simulink model "DC"  (R2016b)
settings: Solver=ode4  StartTime=0.0  StopTime=Inf  FixedStep=0.005  RelTol=1e-3
settings Model: Creator=ANTO_  LastModifiedBy=ANTO_
settings DebuggingCC: RootOutportRequireBusObject=error  StrictBusMsg=ErrorOnBusTreatedAsVector
settings HardwareCC: ProdBitPerPointer=32  ProdBitPerSizeT=32  ProdBitPerPtrDiffT=32  ProdLargestAtomicInteger=Long  ProdWordSize=32  ProdHWDeviceType=ARM Compatible->ARM 7
settings RTWCC: SystemTargetFile=NIVeriStand_Linux_ARM_32.tlc  TemplateMakefile=NIVeriStand_Linux_ARM_32.tmf  Description=NI Linux Real-Time ARM (32-bit) Target
settings STFCustomTargetCC: TargetLangStandard=C99 (ISO)  MatFileLogging=on  MATLABClassNameForMDSCustomization=Simulink.SoftwareTarget.TargetSpecificTriggerConfigurationBase  SystemTargetFile=NIVeriStand_Linux_ARM_32.tlc

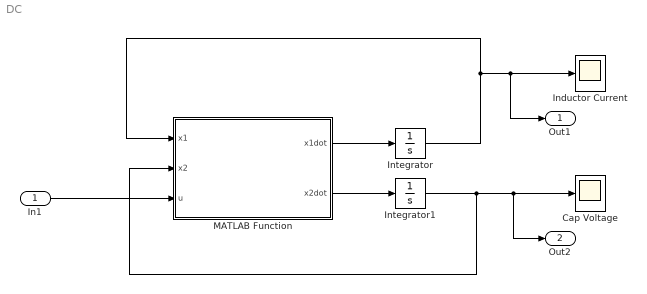
== system DC ==
  In1 : Inport
  Cap Voltage : Scope
  Inductor Current : Scope
  Integrator : Integrator  InitialCondition=0.7
  Integrator1 : Integrator  InitialCondition=5.4
  MATLAB Function : MATLAB Function  TreatAsAtomicUnit=on
  Out1 : Outport
  Out2 : Outport  Port=2
  wires:
  MATLAB Function/1(x1dot) -> Integrator/1
  MATLAB Function/2(x2dot) -> Integrator1/1
  Integrator/1 -> MATLAB Function/1(x1), Out1/1, Inductor Current/1
  Integrator1/1 -> MATLAB Function/2(x2), Out2/1, Cap Voltage/1
  In1/1 -> MATLAB Function/3(u)

== matlab function DC/MATLAB Function ==
  data: x1 input; x2 input; u input; x1dot output; x2dot output
function [x1dot,x2dot] = Boost_DC_converter(x1,x2,u)

  x = [x1;x2];
  r0=1.0;
  vs = 1.0 ;
  rl = 0.05 ;
  rc = rl / 10 ;
  xl = 3.0 ;
  xc = 70.0 ;

  if(u==1)
    A = [ -rl / xl  0 ;  0  (-1 / xc) * (1 / (r0 + rc)) ] ;
  else
    A = [ (-1 / xl) * (rl + ((r0 * rc) / (r0 + rc)))  ((-1 / xl) * (r0 / (r0 + rc))) / 5 ;
          5 * (r0 / (r0 + rc)) * (1 / xc)  (-1 / xc) * (1 / (r0 + rc)) ];
  end
  b = [(vs / xl) ; 0 ] ;

  dxdt= A*x+b;
  x1dot = dxdt(1);
  x2dot = dxdt(2);
end
